simulink model "soc_rfsoc_proc"  (R2023b)
settings: Solver=FixedStepAuto  StartTime=0.0  StopTime=10.0  RelTol=1e-3  EnableMultiTasking=on
model workspace (MAT data in the model file):
  SrcSel = 0
libraries: prociolib x4
settings Model: Creator=The MathWorks, Inc.  LastModifiedBy=akroh
settings SolverCC: AlgebraicLoopSolver=TrustRegion  PositivePriorityOrder=on
settings DataIOCC: SaveFormat=StructureWithTime  ReturnWorkspaceOutputs=off
settings OptimizationCC: PassReuseOutputArgsAs=Individual arguments  ZeroExternalMemoryAtStartup=off  MaxStackSize=64  EfficientTunableParamExpr=on
settings DebuggingCC: IntegerOverflowMsg=none  ParameterTunabilityLossMsg=error  UnconnectedInputMsg=warning  UnconnectedOutputMsg=warning  UnconnectedLineMsg=warning  ArithmeticOperatorsInVariantConditions=warning
settings HardwareCC: ProdBitPerLong=64  ProdLargestAtomicInteger=LongLong  ProdLargestAtomicFloat=Double  ProdLongLongMode=on  ProdHWDeviceType=ARM Compatible->ARM 64-bit (LP64)  HardwareBoardFeatureSet=SoCBlockset
settings ModelReferenceCC: EnableRefExpFcnMdlSchedulingChecks=on  ModelReferenceNumInstancesAllowed=Single
settings SFSimCC: SimUseLocalCustomCode=off
settings RTWCC: Description=Embedded Coder  SystemTargetFile=ert.tlc  HardwareBoard=Xilinx Zynq UltraScale+ RFSoC ZCU111 Evaluation Kit  TLCOptions="-aInlineSetEventsForThisBaseRateFcn=TLC_FALSE -aSuppressMultiTaskScheduler=TLC_FALSE  -aRateBasedStepFcn=0"  GenCodeOnly=on  TemplateMakefile=ert_default_tmf  GenerateReport=on  RTWUseLocalCustomCode=off  Toolchain=Linaro AArch64 Linux v6.3.1  IncludeHyperlinkInReport=on  LaunchReport=on  GenerateTraceInfo=on  GenerateTraceReport=on  GenerateTraceReportSl=on  GenerateTraceReportSf=on  GenerateTraceReportEml=on  DLArmComputeVersion=19.05
settings CodeAppCC: ForceParamTrailComments=on  IgnoreCustomStorageClasses=off  OperatorAnnotations=on  SimulinkDataObjDesc=on  SFDataObjDesc=on  InsertBlockDesc=on

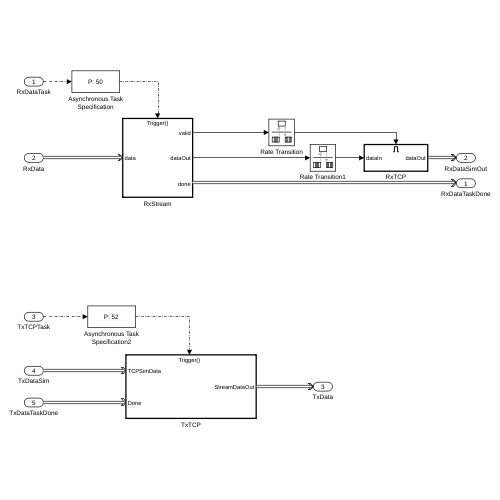
[thumbnail: Simulink's stored preview of the top-level diagram]
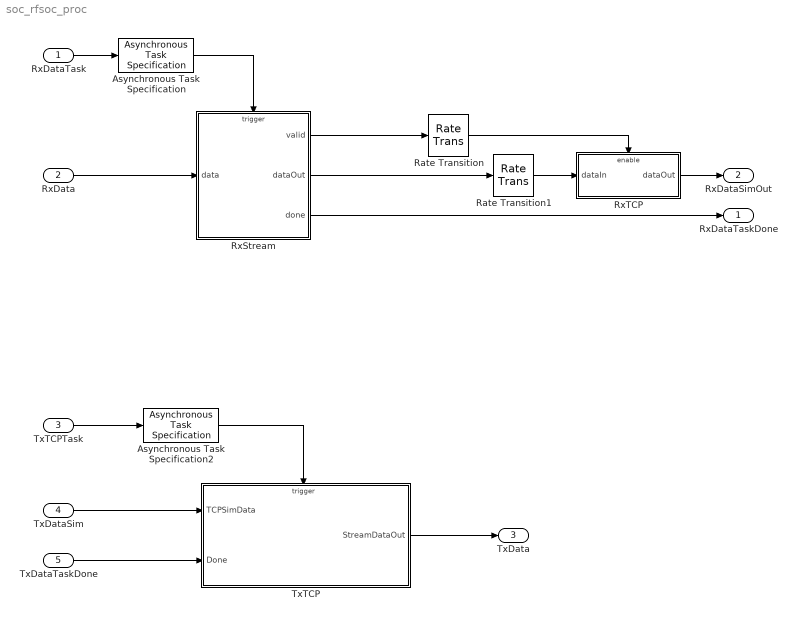
== system soc_rfsoc_proc ==
  RxDataTask : Inport  OutputFunctionCall=on
  RxData : Inport  OutputPortMessageModes=m  Port=2  OutDataTypeStr=SoCData  BusOutputAsStruct=on
  TxTCPTask : Inport  Port=3  OutputFunctionCall=on
  TxDataSim : Inport  OutputPortMessageModes=m  Port=4  OutDataTypeStr=SoCData  BusOutputAsStruct=on
  TxDataTaskDone : Inport  OutputPortMessageModes=m  Port=5
  Asynchronous Task Specification : AsynchronousTaskSpecification  TaskPriority=50
  Asynchronous Task Specification2 : AsynchronousTaskSpecification  TaskPriority=52
  Rate Transition : RateTransition  Deterministic=off  OutPortSampleTime=1e-3
  Rate Transition1 : RateTransition  Deterministic=off  OutPortSampleTime=1e-3
  RxStream : Subsystem  TreatAsAtomicUnit=on
  RxTCP : Subsystem  TreatAsAtomicUnit=on
  TxTCP : Subsystem  TreatAsAtomicUnit=on
  RxDataTaskDone : Outport  InputPortMessageModes=m  VectorParamsAs1DForOutWhenUnconnected=off  BusOutputAsStruct=on
  RxDataSimOut : Outport  InputPortMessageModes=m  Port=2  VectorParamsAs1DForOutWhenUnconnected=off
  TxData : Outport  InputPortMessageModes=m  Port=3  VectorParamsAs1DForOutWhenUnconnected=off
  wires:
  RxDataTask/1 -> Asynchronous Task Specification/1
  RxData/1 -> RxStream/1(data)
  RxStream/3(done) -> RxDataTaskDone/1
  RxStream/2(dataOut) -> Rate Transition1/1
  Asynchronous Task Specification/1 -> RxStream/Trigger
  RxStream/1(valid) -> Rate Transition/1
  RxTCP/1(dataOut) -> RxDataSimOut/1
  TxDataSim/1 -> TxTCP/1(TCPSimData)
  TxDataTaskDone/1 -> TxTCP/2(Done)
  Rate Transition/1 -> RxTCP/Enable
  Rate Transition1/1 -> RxTCP/1(dataIn)
  TxTCPTask/1 -> Asynchronous Task Specification2/1
  Asynchronous Task Specification2/1 -> TxTCP/Trigger
  TxTCP/1(StreamDataOut) -> TxData/1

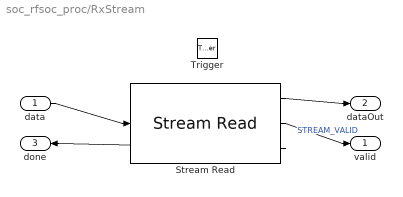
== system soc_rfsoc_proc/RxStream ==
  data : Inport
  Trigger : TriggerPort  TriggerType=function-call  VariantControl=Variant  PortDimensions=1
  Stream Read : prociolib/Stream Read  DeviceName=ip:s2mm  OutDataTypeStr=uint32  SamplesPerFrame=FrameSize  NumberOfBuffers=NumBuffers  EnableEvent=on  SampleTime=-1
  valid : Outport
  dataOut : Outport  Port=2  VectorParamsAs1DForOutWhenUnconnected=off
  done : Outport  Port=3  VectorParamsAs1DForOutWhenUnconnected=off
  wires:
  data/1 -> Stream Read/1
  Stream Read/3 -> done/1
  Stream Read/1 -> dataOut/1
  Stream Read/2 -> valid/1  "STREAM_VALID"

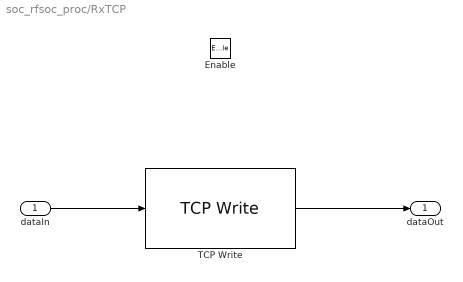
== system soc_rfsoc_proc/RxTCP ==
  dataIn : Inport
  Enable : EnablePort
  TCP Write : prociolib/TCP Write  NetworkRole=Server  RemoteAddress=127.0.0.1  RemotePort=25000  LocalPort=12002  ByteOrder=LittleEndian  OutputStatus=off  hoistedMaskSrc=Variant/CODEGEN/TCP Write
  dataOut : Outport
  wires:
  dataIn/1 -> TCP Write/1
  TCP Write/1 -> dataOut/1

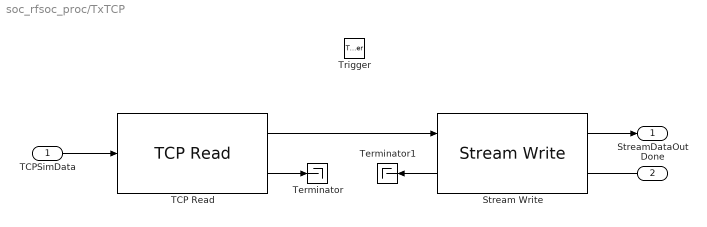
== system soc_rfsoc_proc/TxTCP ==
  TCPSimData : Inport
  Done : Inport  Port=2
  Trigger : TriggerPort  TriggerType=function-call  VariantControl=Variant  PortDimensions=1
  Stream Write : prociolib/Stream Write  DeviceName=ip:mm2s  NumberOfBuffers=NumBuffers  EnableEvent=on
  TCP Read : prociolib/TCP Read  NetworkRole=Server  RemoteAddress=127.0.0.1  RemotePort=25000  LocalPort=12001  DataType=uint32  DataLength=FrameSize  ByteOrder=LittleEndian  EnableEvent=on  OutputVarSizeSignal=off  OutputStatus=off  SampleTime=-1  hoistedMaskSrc=Variant/CODEGEN/TCP Read
  Terminator : Terminator
  Terminator1 : Terminator
  StreamDataOut : Outport
  wires:
  TCPSimData/1 -> TCP Read/1
  TCP Read/2 -> Terminator/1
  Stream Write/1 -> StreamDataOut/1
  Done/1 -> Stream Write/2
  Stream Write/2 -> Terminator1/1
  TCP Read/1 -> Stream Write/1
